simulink model "probelm_4"  (R2020a)
settings: Solver=VariableStepAuto  StartTime=0.0  StopTime=10  RelTol=1e-3
model workspace (MAT data in the model file):
  J = 3.2284e-06
  L = 2.75e-06
  R = 4
  b = 3.5077e-06
  kd = 0.125612262604
  ke = 0.0274
  ki = 372.024702765
  kp = 15.1715978788
  kt = 0.0274
settings Model: Creator=Shubham Singh Rathor  LastModifiedBy=Shubham Singh Rathor

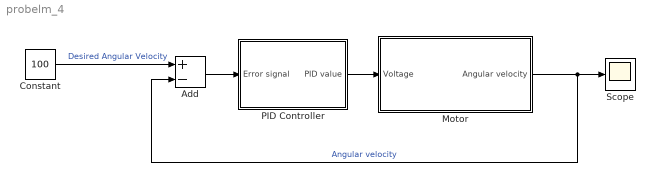
== system probelm_4 ==
  Add : Sum  Inputs=+-
  Constant : Constant  Value=100
  Motor : Subsystem
  PID Controller : Subsystem
  Scope : Scope
  wires:
  Motor/1(Angular velocity) -> Add/2, Scope/1  "Angular velocity"
  Constant/1 -> Add/1  "Desired Angular Velocity"
  Add/1 -> PID Controller/1(Error signal)
  PID Controller/1(PID value) -> Motor/1(Voltage)

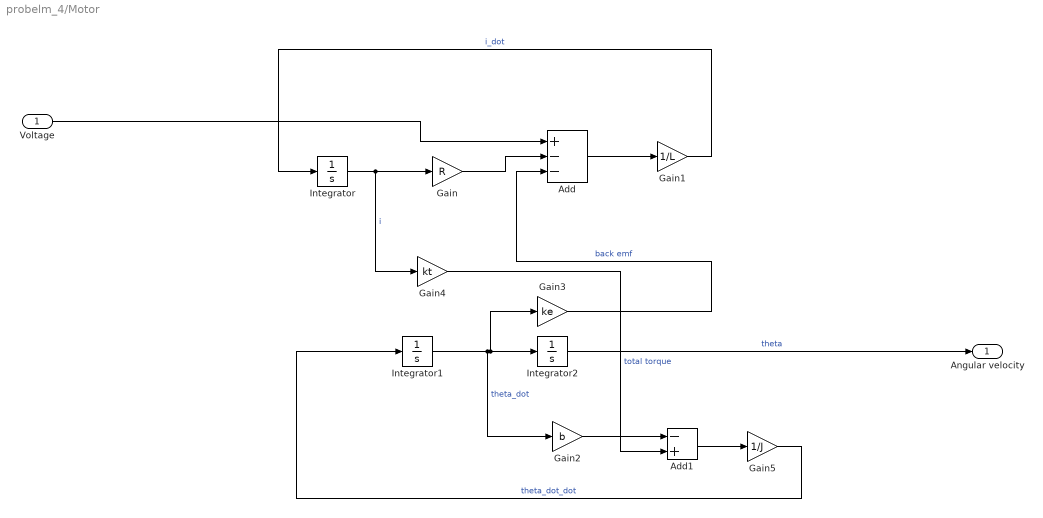
== system probelm_4/Motor ==
  Voltage : Inport
  Add : Sum  Inputs=+--
  Add1 : Sum  Inputs=-+
  Gain : Gain  Gain=R
  Gain1 : Gain  Gain=1/L
  Gain2 : Gain  Gain=b
  Gain3 : Gain  Gain=ke
  Gain4 : Gain  Gain=kt
  Gain5 : Gain  Gain=1/J
  Integrator : Integrator
  Integrator1 : Integrator
  Integrator2 : Integrator
  Angular velocity : Outport
  wires:
  Integrator1/1 -> Gain2/1, Gain3/1, Integrator2/1  "theta_dot"
  Gain5/1 -> Integrator1/1  "theta_dot_dot"
  Gain/1 -> Add/2
  Add1/1 -> Gain5/1
  Integrator/1 -> Gain4/1, Gain/1  "i"
  Gain2/1 -> Add1/1
  Gain4/1 -> Add1/2  "total torque"
  Gain3/1 -> Add/3  "back emf"
  Add/1 -> Gain1/1
  Gain1/1 -> Integrator/1  "i_dot"
  Integrator2/1 -> Angular velocity/1  "theta"
  Voltage/1 -> Add/1

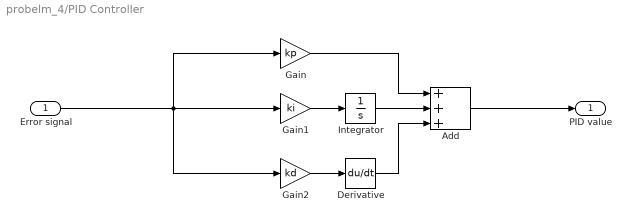
== system probelm_4/PID Controller ==
  Error signal : Inport
  Add : Sum  Inputs=+++
  Derivative : Derivative  CoefficientInTFapproximation=1575.03337415742
  Gain : Gain  Gain=kp
  Gain1 : Gain  Gain=ki
  Gain2 : Gain  Gain=kd
  Integrator : Integrator
  PID value : Outport
  wires:
  Error signal/1 -> Gain2/1, Gain1/1, Gain/1
  Gain/1 -> Add/1
  Gain2/1 -> Derivative/1
  Integrator/1 -> Add/2
  Add/1 -> PID value/1
  Gain1/1 -> Integrator/1
  Derivative/1 -> Add/3
